simulink model "AirCooledDataCenterTemperatureProfile"  (R2025b)
settings: Solver=daessc  StartTime=0.0  StopTime=24*3600  MaxStep=1  RelTol=1e-3  AbsTol=1e-3
PreLoadFcn:
  | if ~exist("airCooledDataCenter")
  |     setModelParam;
  | end
undefined symbols (not defined in the file or in its folder): airCooledDataCenter, DiscIntNeverNeededParam, value
libraries: fl_lib x166, nesl_utility x25, datacenter_lib x24, simulink_extras x9
(part 2 of 4)

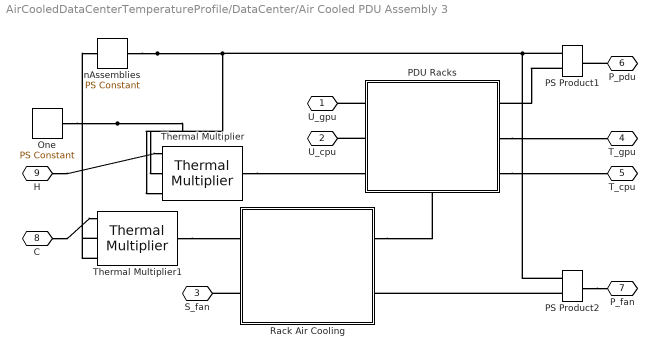
== system AirCooledDataCenterTemperatureProfile/DataCenter/Air Cooled PDU Assembly 3 ==
  One : fl_lib/Physical Signals/Sources/PS Constant  constant=1
  PDU Racks : Subsystem  mask{nTrays=nTrays, nRacks=nRacks, trayMass=trayMass, trayCp=trayCp, trayThermalR=trayThermalR, nGPU=nGPU, gpuTDPperDie=gpuTDPperDie, gpuIdlePower=gpuIdlePower, gpuHBMpower=gpuHBMpower, gpuExponent=gpuExponent, gpuHBMutil=gpuHBMutil, gpuLeakage=gpuLeakage, gpuNominalDieT=gpuNominalDieT, gpuDieThermalC=gpuDieThermalC, gpuHeatSinkR=gpuHeatSinkR, gpuSurfArea=gpuSurfArea, gpuAmbientR=gpuAmbientR, nCPU=nCPU, cpuTDPperSocket=cpuTDPperSocket, cpuIdlePower=cpuIdlePower, cpuExponent=cpuExponent, cpuLeakage=cpuLeakage, cpuNominalDieT=cpuNominalDieT, cpuDieThermalC=cpuDieThermalC, cpuHeatSinkR=cpuHeatSinkR, cpuSurfArea=cpuSurfArea, cpuAmbientR=cpuAmbientR, initialT=initialT, htc=htc}
      mask prompts: nTrays "Number of IT trays per rack (-)"; nRacks "Number of racks (-)"; trayMass "Tray mass (kg)"; trayCp "Tray specific heat capacity (J/kg*K)"; trayThermalR "Tray to external thermal resistance (K/W)"; nGPU "Number of GPU per tray (-)"; gpuTDPperDie "GPU TDP per die (W)"; gpuIdlePower "GPU idle power (W)"; gpuHBMpower "HBM power per GPU (W)"; gpuExponent "GPU power utilization exponent (-)"; gpuHBMutil "HBM utilization as fraction of compute utilization (-)"; gpuLeakage "Leakage increase per K above nominal temperature (W/K)"; gpuNominalDieT "Nominal die temperature at TDP (K)"; gpuDieThermalC "GPU die thermal capacitance (J/K)"; gpuHeatSinkR "GPU die-heat-sink thermal resistance (K/W)"; gpuSurfArea "Surface area per die for ambient heat transfer (m^2)"; gpuAmbientR "GPU die-ambient thermal resistance (K/W)"; nCPU "Number of CPU per tray (-)"; cpuTDPperSocket "CPU TDP per socket (W)"; cpuIdlePower "CPU idle power per socket (W)"; cpuExponent "CPU power utilization exponent (-)"; cpuLeakage "Leakage increase per K above nominal temperature (W/K)"; cpuNominalDieT "Nominal die temperature at TDP (K)"; cpuDieThermalC "CPU die thermal capacitance (J/K)"; cpuHeatSinkR "CPU die-heat-sink thermal resistance (K/W)"; cpuSurfArea "Surface area per die for ambient heat transfer (m^2)"; cpuAmbientR "CPU die-ambient thermal resistance (K/W)"; initialT "Initial temperature (K)"; htc "Heat transfer coefficient to ambient (W/m^2.K)"
      settings: CopyFcn=set_param(gcbh,'LinkStatus','none');  PortSchema="{\"entries\":[{\"content\":{\"sides\":[{\"content\":{\"connectorIds\":[\"LConn1\",\"LConn2\",\"LConn3\"]},\"type\":\"ConnectorPlacement.EquallySpacedRectSide\",\"uuid\":\"1a9a884a-dab1-4495-bf62-c6b2de6c1039\"},{\"content\":{\"connectorIds\":[\"RConn1\",\"RConn2\",\"RConn3\"],\"side\":\"RIGHT\"},\"type\":\"ConnectorPlacement.EquallySpacedRectSide\",\"uuid\":\"05c53434-51c1-4fee-b885-c321dcda8b6b\"},{\"content\":{\"side\":\"TOP\"},\"type\":\"ConnectorPlacement.EquallySpacedRectSide\",\"uuid\":\"c7b5c534-d596-4858-a133-27f005e6c9d4\"},{\"content\":{\"connectorIds\":[\"RConn4\"],\"side\":\"BOTTOM\"},\"type\":\"ConnectorPlacement.EquallySpacedRectSide\",\"uuid\":\"693f3c99-4296-4d86-bfcc-da753d3e576f\"}]},\"type\":\"ConnectorPlacement.EquallySpacedConnector\",\"uuid\":\"ed91c467-c4d0-403f-af16-bac0257594fd\"}],\"packageUris\":[\"http://schema.mathworks.com/mf0/Connector/R2020b\"],\"version\":\"1.0\"}"
      mask Help: web("DocumentationPDURacks.html")
      mask DialogControl Container10 Prompt: PDU Racks
      mask DialogControl getRatingButton Prompt: Get Rating
      mask DialogControl Container9 Prompt: IT Tray
      mask DialogControl Container6 Prompt: GPU
      mask DialogControl Container7 Prompt: CPU
      mask DialogControl Container8 Prompt: Initial Conditions
      mask Display: image('icon_PDURacks.png');
  PS Product1 : fl_lib/Physical Signals/Functions/PS Product
  PS Product2 : fl_lib/Physical Signals/Functions/PS Product
  Rack Air Cooling : Subsystem  mask{nFans=nFans, flowVec=flowVec, prDropVec=prDropVec, fanEffVec=fanEffVec, fluidDen=1.28, fluidCp=1005}
      mask prompts: nFans "Number of fans (-)"; flowVec "Fan flow rate vector (m^3/s)"; prDropVec "Pressure drop vector (Pa)"; fanEffVec "Fan efficiency vector (-)"; fluidDen "Fluid density (kg/m^3)"; fluidCp "Fluid heat capacity (J/(Kg*K))"
      settings: CopyFcn=set_param(gcbh,'LinkStatus','none');
      mask Help: web("DocumentationRackAirCooling.html")
      mask DialogControl Container3 Prompt: Fans
      mask DialogControl Container4 Prompt: Fluid Properties
      mask Display: image('icon_PDUfanCooling.png');
  Thermal Multiplier : datacenter_lib/Thermal Multiplier
      settings: InternalSimscapePortConfiguration="{\"Bottom\":[],\"Left\":[{\"id\":\"A\",\"label\":\"A\",\"type\":\"foundation.thermal.thermal\"}],\"Right\":[{\"id\":\"B\",\"label\":\"B\",\"type\":\"foundation.thermal.thermal\"}],\"Top\":[{\"id\":\"Na\",\"label\":\"Na\",\"type\":\"input\"},{\"id\":\"Nb\",\"label\":\"Nb\",\"type\":\"input\"}]}"
  Thermal Multiplier1 : datacenter_lib/Thermal Multiplier
      settings: InternalSimscapePortConfiguration="{\"Bottom\":[],\"Left\":[{\"id\":\"A\",\"label\":\"A\",\"type\":\"foundation.thermal.thermal\"}],\"Right\":[{\"id\":\"B\",\"label\":\"B\",\"type\":\"foundation.thermal.thermal\"}],\"Top\":[{\"id\":\"Na\",\"label\":\"Na\",\"type\":\"input\"},{\"id\":\"Nb\",\"label\":\"Nb\",\"type\":\"input\"}]}"
  nAssemblies : fl_lib/Physical Signals/Sources/PS Constant  constant=nAssembly
  U_gpu : PMIOPort  Side=Left
  U_cpu : PMIOPort  Port=2  Side=Left
  S_fan : PMIOPort  Port=3  Side=Left
  T_gpu : PMIOPort  Port=4  Side=Right
  T_cpu : PMIOPort  Port=5  Side=Right
  P_pdu : PMIOPort  Port=6  Side=Right
  P_fan : PMIOPort  Port=7  Side=Right
  C : PMIOPort  Port=8  Side=Left
  H : PMIOPort  Port=9  Side=Right
  connections:
  C/RConn1 -- Thermal Multiplier1/LConn1
  H/RConn1 -- Thermal Multiplier/LConn1
  Thermal Multiplier1/RConn1 -- Rack Air Cooling/LConn1
  PS Product2/LConn2 -- Rack Air Cooling/RConn2
  PS Product2/RConn1 -- P_fan/RConn1
  PS Product1/LConn2 -- PDU Racks/RConn1
  P_pdu/RConn1 -- PS Product1/RConn1
  Thermal Multiplier/LConn2 -- Thermal Multiplier1/LConn2 -- One/RConn1
  Thermal Multiplier/LConn3 -- PS Product2/LConn1 -- PS Product1/LConn1 -- Thermal Multiplier1/LConn3 -- nAssemblies/RConn1
  Thermal Multiplier/RConn1 -- PDU Racks/LConn3
  PDU Racks/LConn1 -- U_gpu/RConn1
  Rack Air Cooling/LConn2 -- S_fan/RConn1
  PDU Racks/RConn2 -- T_gpu/RConn1
  PDU Racks/LConn2 -- U_cpu/RConn1
  PDU Racks/RConn3 -- T_cpu/RConn1
  Rack Air Cooling/RConn1 -- PDU Racks/RConn4

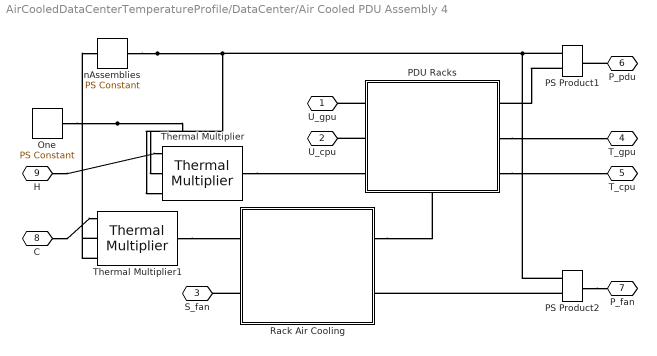
== system AirCooledDataCenterTemperatureProfile/DataCenter/Air Cooled PDU Assembly 4 ==
  One : fl_lib/Physical Signals/Sources/PS Constant  constant=1
  PDU Racks : Subsystem  mask{nTrays=nTrays, nRacks=nRacks, trayMass=trayMass, trayCp=trayCp, trayThermalR=trayThermalR, nGPU=nGPU, gpuTDPperDie=gpuTDPperDie, gpuIdlePower=gpuIdlePower, gpuHBMpower=gpuHBMpower, gpuExponent=gpuExponent, gpuHBMutil=gpuHBMutil, gpuLeakage=gpuLeakage, gpuNominalDieT=gpuNominalDieT, gpuDieThermalC=gpuDieThermalC, gpuHeatSinkR=gpuHeatSinkR, gpuSurfArea=gpuSurfArea, gpuAmbientR=gpuAmbientR, nCPU=nCPU, cpuTDPperSocket=cpuTDPperSocket, cpuIdlePower=cpuIdlePower, cpuExponent=cpuExponent, cpuLeakage=cpuLeakage, cpuNominalDieT=cpuNominalDieT, cpuDieThermalC=cpuDieThermalC, cpuHeatSinkR=cpuHeatSinkR, cpuSurfArea=cpuSurfArea, cpuAmbientR=cpuAmbientR, initialT=initialT, htc=htc}
      mask prompts: nTrays "Number of IT trays per rack (-)"; nRacks "Number of racks (-)"; trayMass "Tray mass (kg)"; trayCp "Tray specific heat capacity (J/kg*K)"; trayThermalR "Tray to external thermal resistance (K/W)"; nGPU "Number of GPU per tray (-)"; gpuTDPperDie "GPU TDP per die (W)"; gpuIdlePower "GPU idle power (W)"; gpuHBMpower "HBM power per GPU (W)"; gpuExponent "GPU power utilization exponent (-)"; gpuHBMutil "HBM utilization as fraction of compute utilization (-)"; gpuLeakage "Leakage increase per K above nominal temperature (W/K)"; gpuNominalDieT "Nominal die temperature at TDP (K)"; gpuDieThermalC "GPU die thermal capacitance (J/K)"; gpuHeatSinkR "GPU die-heat-sink thermal resistance (K/W)"; gpuSurfArea "Surface area per die for ambient heat transfer (m^2)"; gpuAmbientR "GPU die-ambient thermal resistance (K/W)"; nCPU "Number of CPU per tray (-)"; cpuTDPperSocket "CPU TDP per socket (W)"; cpuIdlePower "CPU idle power per socket (W)"; cpuExponent "CPU power utilization exponent (-)"; cpuLeakage "Leakage increase per K above nominal temperature (W/K)"; cpuNominalDieT "Nominal die temperature at TDP (K)"; cpuDieThermalC "CPU die thermal capacitance (J/K)"; cpuHeatSinkR "CPU die-heat-sink thermal resistance (K/W)"; cpuSurfArea "Surface area per die for ambient heat transfer (m^2)"; cpuAmbientR "CPU die-ambient thermal resistance (K/W)"; initialT "Initial temperature (K)"; htc "Heat transfer coefficient to ambient (W/m^2.K)"
      settings: CopyFcn=set_param(gcbh,'LinkStatus','none');  PortSchema="{\"entries\":[{\"content\":{\"sides\":[{\"content\":{\"connectorIds\":[\"LConn1\",\"LConn2\",\"LConn3\"]},\"type\":\"ConnectorPlacement.EquallySpacedRectSide\",\"uuid\":\"1a9a884a-dab1-4495-bf62-c6b2de6c1039\"},{\"content\":{\"connectorIds\":[\"RConn1\",\"RConn2\",\"RConn3\"],\"side\":\"RIGHT\"},\"type\":\"ConnectorPlacement.EquallySpacedRectSide\",\"uuid\":\"05c53434-51c1-4fee-b885-c321dcda8b6b\"},{\"content\":{\"side\":\"TOP\"},\"type\":\"ConnectorPlacement.EquallySpacedRectSide\",\"uuid\":\"c7b5c534-d596-4858-a133-27f005e6c9d4\"},{\"content\":{\"connectorIds\":[\"RConn4\"],\"side\":\"BOTTOM\"},\"type\":\"ConnectorPlacement.EquallySpacedRectSide\",\"uuid\":\"693f3c99-4296-4d86-bfcc-da753d3e576f\"}]},\"type\":\"ConnectorPlacement.EquallySpacedConnector\",\"uuid\":\"ed91c467-c4d0-403f-af16-bac0257594fd\"}],\"packageUris\":[\"http://schema.mathworks.com/mf0/Connector/R2020b\"],\"version\":\"1.0\"}"
      mask Help: web("DocumentationPDURacks.html")
      mask DialogControl Container10 Prompt: PDU Racks
      mask DialogControl getRatingButton Prompt: Get Rating
      mask DialogControl Container9 Prompt: IT Tray
      mask DialogControl Container6 Prompt: GPU
      mask DialogControl Container7 Prompt: CPU
      mask DialogControl Container8 Prompt: Initial Conditions
      mask Display: image('icon_PDURacks.png');
  PS Product1 : fl_lib/Physical Signals/Functions/PS Product
  PS Product2 : fl_lib/Physical Signals/Functions/PS Product
  Rack Air Cooling : Subsystem  mask{nFans=nFans, flowVec=flowVec, prDropVec=prDropVec, fanEffVec=fanEffVec, fluidDen=1.28, fluidCp=1005}
      mask prompts: nFans "Number of fans (-)"; flowVec "Fan flow rate vector (m^3/s)"; prDropVec "Pressure drop vector (Pa)"; fanEffVec "Fan efficiency vector (-)"; fluidDen "Fluid density (kg/m^3)"; fluidCp "Fluid heat capacity (J/(Kg*K))"
      settings: CopyFcn=set_param(gcbh,'LinkStatus','none');
      mask Help: web("DocumentationRackAirCooling.html")
      mask DialogControl Container3 Prompt: Fans
      mask DialogControl Container4 Prompt: Fluid Properties
      mask Display: image('icon_PDUfanCooling.png');
  Thermal Multiplier : datacenter_lib/Thermal Multiplier
      settings: InternalSimscapePortConfiguration="{\"Bottom\":[],\"Left\":[{\"id\":\"A\",\"label\":\"A\",\"type\":\"foundation.thermal.thermal\"}],\"Right\":[{\"id\":\"B\",\"label\":\"B\",\"type\":\"foundation.thermal.thermal\"}],\"Top\":[{\"id\":\"Na\",\"label\":\"Na\",\"type\":\"input\"},{\"id\":\"Nb\",\"label\":\"Nb\",\"type\":\"input\"}]}"
  Thermal Multiplier1 : datacenter_lib/Thermal Multiplier
      settings: InternalSimscapePortConfiguration="{\"Bottom\":[],\"Left\":[{\"id\":\"A\",\"label\":\"A\",\"type\":\"foundation.thermal.thermal\"}],\"Right\":[{\"id\":\"B\",\"label\":\"B\",\"type\":\"foundation.thermal.thermal\"}],\"Top\":[{\"id\":\"Na\",\"label\":\"Na\",\"type\":\"input\"},{\"id\":\"Nb\",\"label\":\"Nb\",\"type\":\"input\"}]}"
  nAssemblies : fl_lib/Physical Signals/Sources/PS Constant  constant=nAssembly
  U_gpu : PMIOPort  Side=Left
  U_cpu : PMIOPort  Port=2  Side=Left
  S_fan : PMIOPort  Port=3  Side=Left
  T_gpu : PMIOPort  Port=4  Side=Right
  T_cpu : PMIOPort  Port=5  Side=Right
  P_pdu : PMIOPort  Port=6  Side=Right
  P_fan : PMIOPort  Port=7  Side=Right
  C : PMIOPort  Port=8  Side=Left
  H : PMIOPort  Port=9  Side=Right
  connections:
  C/RConn1 -- Thermal Multiplier1/LConn1
  H/RConn1 -- Thermal Multiplier/LConn1
  Thermal Multiplier1/RConn1 -- Rack Air Cooling/LConn1
  PS Product2/LConn2 -- Rack Air Cooling/RConn2
  PS Product2/RConn1 -- P_fan/RConn1
  PS Product1/LConn2 -- PDU Racks/RConn1
  P_pdu/RConn1 -- PS Product1/RConn1
  Thermal Multiplier/LConn2 -- Thermal Multiplier1/LConn2 -- One/RConn1
  Thermal Multiplier/LConn3 -- PS Product2/LConn1 -- PS Product1/LConn1 -- Thermal Multiplier1/LConn3 -- nAssemblies/RConn1
  Thermal Multiplier/RConn1 -- PDU Racks/LConn3
  PDU Racks/LConn1 -- U_gpu/RConn1
  Rack Air Cooling/LConn2 -- S_fan/RConn1
  PDU Racks/RConn2 -- T_gpu/RConn1
  PDU Racks/LConn2 -- U_cpu/RConn1
  PDU Racks/RConn3 -- T_cpu/RConn1
  Rack Air Cooling/RConn1 -- PDU Racks/RConn4

== system AirCooledDataCenterTemperatureProfile/DataCenter/Lumped Room ==
  Controlled Temperature Source : fl_lib/Thermal/Thermal Sources/Controlled Temperature Source
  Convective Heat Transfer : fl_lib/Thermal/Thermal Elements/Convective Heat Transfer  thermal_type=foundation.enum.constant_variable.constant  area=len*wid m^2  heat_tr_coeff=htc W/(K*m^2)  min_heat_tr_coeff=1e-3 W/(K*m^2)  T_specify=off  T_priority=None  T=0 K  T_nominal_specify=off  T_nominal_value=1  T_nominal_unit=K  Q_specify=off  Q_priority=None  Q=0 W  Q_nominal_specify=off  Q_nominal_value=1  Q_nominal_unit=W
  Convective Heat Transfer1 : fl_lib/Thermal/Thermal Elements/Convective Heat Transfer  thermal_type=foundation.enum.constant_variable.constant  area=4*2*(len+wid)*hgt*pc/100 m^2  heat_tr_coeff=htc W/(K*m^2)  min_heat_tr_coeff=1e-3 W/(K*m^2)  T_specify=off  T_priority=None  T=0 K  T_nominal_specify=off  T_nominal_value=1  T_nominal_unit=K  Q_specify=off  Q_priority=None  Q=0 W  Q_nominal_specify=off  Q_nominal_value=1  Q_nominal_unit=W
  PS-Simulink Converter16 : nesl_utility/PS-Simulink Converter  PhysicalDomain=network_engine_domain  SubClassName=ps_output  LeftPortType=input  RightPortType=output  PseudoPeriodic=off  Frequencies=[]  VectorFormat=inherit  Unit=inherit  AffineConversion=off
  Room air mass : fl_lib/Thermal/Thermal Elements/Thermal Mass  mass_type=foundation.enum.constant_variable.constant  mass=len*wid*hgt*(1-pc/100)*1.28 kg  sp_heat=1005 J/(K*kg)  mass_min=1e-6 kg  num_ports=foundation.enum.numPorts2.two  m_specify=off  m_priority=High  m=1 kg  m_nominal_specify=off  m_nominal_value=1  m_nominal_unit=kg  T_specify=on  T_priority=High  T=iniT K  T_nominal_specify=off  T_nominal_value=1  T_nominal_unit=K  Q_specify=off  Q_priority=None  Q=0 W  Q_nominal_specify=off  Q_nominal_value=1  Q_nominal_unit=W
      settings: InternalSimscapePortConfiguration="{\"Bottom\":[],\"Left\":[{\"id\":\"M\",\"label\":\"\",\"type\":\"foundation.thermal.thermal\"}],\"Right\":[{\"id\":\"N\",\"label\":\"\",\"type\":\"foundation.thermal.thermal\"}],\"Top\":[]}"
  Temperature Sensor : fl_lib/Thermal/Thermal Sensors/Temperature Sensor  temperature_measure=foundation.enum.MeasurementReference.absolute
      settings: InternalSimscapePortConfiguration="{\"Bottom\":[],\"Left\":[{\"id\":\"A\",\"label\":\"A\",\"type\":\"foundation.thermal.thermal\"}],\"Right\":[{\"id\":\"T\",\"label\":\"T\",\"type\":\"output\"}],\"Top\":[]}"
  Thermal Reference : fl_lib/Thermal/Thermal Elements/Thermal Reference
  Ts : PMIOPort  Side=Left
  C : PMIOPort  Port=2  Side=Left
  H : PMIOPort  Port=3  Side=Right
  Amb : PMIOPort  Port=4  Side=Right
  Tr : Outport
  wires:
  PS-Simulink Converter16/1 -> Tr/1  "Room T"
  connections:
  Temperature Sensor/LConn1 -- Room air mass/LConn1
  Thermal Reference/LConn1 -- Controlled Temperature Source/RConn2
  Temperature Sensor/RConn1 -- Controlled Temperature Source/RConn1 -- PS-Simulink Converter16/LConn1
  Ts/RConn1 -- Convective Heat Transfer/LConn1
  C/RConn1 -- Controlled Temperature Source/LConn1
  Convective Heat Transfer/RConn1 -- Room air mass/RConn1 -- Amb/RConn1 -- Convective Heat Transfer1/LConn1
  Convective Heat Transfer1/RConn1 -- H/RConn1

== system AirCooledDataCenterTemperatureProfile/Fan Speed Control/Subsystem4 ==
  PS Concatenate : fl_lib/Physical Signals/Functions/PS Concatenate  catColumns=true
      settings: InternalSimscapePortConfiguration="{\"Bottom\":[],\"Left\":[{\"id\":\"I1\",\"label\":\"\",\"type\":\"input\"},{\"id\":\"I2\",\"label\":\"\",\"type\":\"input\"}],\"Right\":[{\"id\":\"O\",\"label\":\"\",\"type\":\"output\"}],\"Top\":[]}"
  PS Concatenate1 : fl_lib/Physical Signals/Functions/PS Concatenate  catColumns=true
      settings: InternalSimscapePortConfiguration="{\"Bottom\":[],\"Left\":[{\"id\":\"I1\",\"label\":\"\",\"type\":\"input\"},{\"id\":\"I2\",\"label\":\"\",\"type\":\"input\"}],\"Right\":[{\"id\":\"O\",\"label\":\"\",\"type\":\"output\"}],\"Top\":[]}"
  PS Concatenate2 : fl_lib/Physical Signals/Functions/PS Concatenate  catColumns=true
      settings: InternalSimscapePortConfiguration="{\"Bottom\":[],\"Left\":[{\"id\":\"I1\",\"label\":\"\",\"type\":\"input\"},{\"id\":\"I2\",\"label\":\"\",\"type\":\"input\"}],\"Right\":[{\"id\":\"O\",\"label\":\"\",\"type\":\"output\"}],\"Top\":[]}"
  S4 : PMIOPort  Side=Left
  S3 : PMIOPort  Port=2  Side=Left
  S2 : PMIOPort  Port=3  Side=Left
  S1 : PMIOPort  Port=4  Side=Left
  F : PMIOPort  Port=5  Side=Right
  connections:
  PS Concatenate2/LConn2 -- S4/RConn1
  PS Concatenate/LConn2 -- S2/RConn1
  PS Concatenate1/LConn1 -- PS Concatenate/RConn1
  PS Concatenate2/LConn1 -- PS Concatenate1/RConn1
  PS Concatenate1/LConn2 -- S3/RConn1
  F/RConn1 -- PS Concatenate2/RConn1
  PS Concatenate/LConn1 -- S1/RConn1

== system AirCooledDataCenterTemperatureProfile/Fan Speed Control/Subsystem5 ==
  T : Inport
  D1 : BusSelector  OutputSignals=D1.Max,D1.Min
  D2 : BusSelector  OutputSignals=D2.Max,D2.Min
  D3 : BusSelector  OutputSignals=D3.Max,D3.Min
  D4 : BusSelector  OutputSignals=D4.Max,D4.Min
  Subsystem : Subsystem  mask{Ts=measDelay, uppT=upperT, lowT=lowerT}
      mask prompts: Ts "Measurement delay (s)"; uppT "Upper limit temperature (K)"; lowT "Lower limit temperature (K)"
      settings: PortSchema="{\"entries\":[{\"content\":{\"sides\":[{\"content\":{\"connectorIds\":[\"LConn1\"]},\"type\":\"ConnectorPlacement.EquallySpacedRectSide\",\"uuid\":\"76a0f47d-e2da-464e-af47-d1de2c0a2775\"},{\"content\":{\"connectorIds\":[\"In1\",\"In2\"],\"side\":\"RIGHT\"},\"type\":\"ConnectorPlacement.EquallySpacedRectSide\",\"uuid\":\"4720b8d8-bdaf-4068-88d8-7e817175b798\"},{\"content\":{\"side\":\"TOP\"},\"type\":\"ConnectorPlacement.EquallySpacedRectSide\",\"uuid\":\"0c4cf0ed-7be6-4add-afae-556b60096d13\"}]},\"type\":\"ConnectorPlacement.EquallySpacedConnector\",\"uuid\":\"5d672270-c8d8-4cc8-adff-c30d9f578126\"}],\"packageUris\":[\"http://schema.mathworks.com/mf0/Connector/R2020b\"],\"version\":\"1.0\"}"
  Subsystem1 : Subsystem  mask{Ts=measDelay, uppT=upperT, lowT=lowerT}
      mask prompts: Ts "Measurement delay (s)"; uppT "Upper limit temperature (K)"; lowT "Lower limit temperature (K)"
      settings: PortSchema="{\"entries\":[{\"content\":{\"sides\":[{\"content\":{\"connectorIds\":[\"LConn1\"]},\"type\":\"ConnectorPlacement.EquallySpacedRectSide\",\"uuid\":\"76a0f47d-e2da-464e-af47-d1de2c0a2775\"},{\"content\":{\"connectorIds\":[\"In1\",\"In2\"],\"side\":\"RIGHT\"},\"type\":\"ConnectorPlacement.EquallySpacedRectSide\",\"uuid\":\"4720b8d8-bdaf-4068-88d8-7e817175b798\"},{\"content\":{\"side\":\"TOP\"},\"type\":\"ConnectorPlacement.EquallySpacedRectSide\",\"uuid\":\"0c4cf0ed-7be6-4add-afae-556b60096d13\"}]},\"type\":\"ConnectorPlacement.EquallySpacedConnector\",\"uuid\":\"5d672270-c8d8-4cc8-adff-c30d9f578126\"}],\"packageUris\":[\"http://schema.mathworks.com/mf0/Connector/R2020b\"],\"version\":\"1.0\"}"
  Subsystem2 : Subsystem  mask{Ts=measDelay, uppT=upperT, lowT=lowerT}
      mask prompts: Ts "Measurement delay (s)"; uppT "Upper limit temperature (K)"; lowT "Lower limit temperature (K)"
      settings: PortSchema="{\"entries\":[{\"content\":{\"sides\":[{\"content\":{\"connectorIds\":[\"LConn1\"]},\"type\":\"ConnectorPlacement.EquallySpacedRectSide\",\"uuid\":\"76a0f47d-e2da-464e-af47-d1de2c0a2775\"},{\"content\":{\"connectorIds\":[\"In1\",\"In2\"],\"side\":\"RIGHT\"},\"type\":\"ConnectorPlacement.EquallySpacedRectSide\",\"uuid\":\"4720b8d8-bdaf-4068-88d8-7e817175b798\"},{\"content\":{\"side\":\"TOP\"},\"type\":\"ConnectorPlacement.EquallySpacedRectSide\",\"uuid\":\"0c4cf0ed-7be6-4add-afae-556b60096d13\"}]},\"type\":\"ConnectorPlacement.EquallySpacedConnector\",\"uuid\":\"5d672270-c8d8-4cc8-adff-c30d9f578126\"}],\"packageUris\":[\"http://schema.mathworks.com/mf0/Connector/R2020b\"],\"version\":\"1.0\"}"
  Subsystem3 : Subsystem  mask{Ts=measDelay, uppT=upperT, lowT=lowerT}
      mask prompts: Ts "Measurement delay (s)"; uppT "Upper limit temperature (K)"; lowT "Lower limit temperature (K)"
      settings: PortSchema="{\"entries\":[{\"content\":{\"sides\":[{\"content\":{\"connectorIds\":[\"LConn1\"]},\"type\":\"ConnectorPlacement.EquallySpacedRectSide\",\"uuid\":\"76a0f47d-e2da-464e-af47-d1de2c0a2775\"},{\"content\":{\"connectorIds\":[\"In1\",\"In2\"],\"side\":\"RIGHT\"},\"type\":\"ConnectorPlacement.EquallySpacedRectSide\",\"uuid\":\"4720b8d8-bdaf-4068-88d8-7e817175b798\"},{\"content\":{\"side\":\"TOP\"},\"type\":\"ConnectorPlacement.EquallySpacedRectSide\",\"uuid\":\"0c4cf0ed-7be6-4add-afae-556b60096d13\"}]},\"type\":\"ConnectorPlacement.EquallySpacedConnector\",\"uuid\":\"5d672270-c8d8-4cc8-adff-c30d9f578126\"}],\"packageUris\":[\"http://schema.mathworks.com/mf0/Connector/R2020b\"],\"version\":\"1.0\"}"
  S1 : PMIOPort  Side=Left
  S2 : PMIOPort  Port=2  Side=Left
  S3 : PMIOPort  Port=3  Side=Left
  S4 : PMIOPort  Port=4  Side=Left
  wires:
  D2/1 -> Subsystem1/1(<Max>)  "<Max>"
  D4/1 -> Subsystem3/1(<Max>)  "<Max>"
  D4/2 -> Subsystem3/2(<Min>)  "<Min>"
  D3/1 -> Subsystem2/1(<Max>)  "<Max>"
  D2/2 -> Subsystem1/2(<Min>)  "<Min>"
  D1/1 -> Subsystem/1(<Max>)  "<Max>"
  D1/2 -> Subsystem/2(<Min>)  "<Min>"
  D3/2 -> Subsystem2/2(<Min>)  "<Min>"
  T/1 -> D4/1, D3/1, D2/1, D1/1
  connections:
  Subsystem2/LConn1 -- S3/RConn1
  Subsystem3/LConn1 -- S4/RConn1
  S1/RConn1 -- Subsystem/LConn1
  Subsystem1/LConn1 -- S2/RConn1

== system AirCooledDataCenterTemperatureProfile/Room HVAC Control/Room HVAC ==
  Tr : Inport
  Ts : Inport  Port=2
  Abs : Abs  SaturateOnIntegerOverflow=off
  Bus Creator : BusCreator  Inputs=2
  Constant2 : Constant  Value=effHeatExchanger/100
  Transfer Fcn (with initial outputs) : simulink_extras/Additional Linear/Transfer Fcn (with initial outputs)  N=[1]  D="[1  tLag]"  Y0=1  U0=0
  air Cp : Constant  Value=1005
  deltaT : Sum  Inputs=+-
  ePower : Product  Inputs=*/
  m_dot_Cp times deltaT : Product  Inputs=3
  mass room air volume : Constant  Value=roomLen*roomWid*roomHt*(1-fracRoomVolDC)*1.28
  S : Outport
  wires:
  Ts/1 -> deltaT/1
  deltaT/1 -> m_dot_Cp times deltaT/3
  Tr/1 -> deltaT/2
  Constant2/1 -> ePower/2
  ePower/1 -> Abs/1
  air Cp/1 -> m_dot_Cp times deltaT/1
  mass room air volume/1 -> m_dot_Cp times deltaT/2
  Abs/1 -> Bus Creator/2  "P"
  Bus Creator/1 -> S/1  "hvac"
  Transfer Fcn (with initial outputs)/1 -> Bus Creator/1, ePower/1  "Q"
  m_dot_Cp times deltaT/1 -> Transfer Fcn (with initial outputs)/1  "Q"

== system AirCooledDataCenterTemperatureProfile/Room HVAC Control/Subsystem ==
  S : Inport
  Bus Selector : BusSelector  OutputSignals=Q,P
  Controlled Heat Flow Rate Source : fl_lib/Thermal/Thermal Sources/Controlled Heat Flow Rate Source
  Simulink-PS Converter : nesl_utility/Simulink-PS Converter  PhysicalDomain=network_engine_domain  SubClassName=ps_input  LeftPortType=input  RightPortType=output  PseudoPeriodic=off  Frequencies=[]  NoiseDistribution=none  NoiseParameters=[]  Unit=J/s  AffineConversion=off  FilteringAndDerivatives=provide  SimscapeFilterOrder=1  InputFilterTimeConstant=0.001  UdotUserProvided=0
  Thermal Reference : fl_lib/Thermal/Thermal Elements/Thermal Reference
  C : PMIOPort  Side=Right
  P : Outport
  wires:
  Bus Selector/1 -> Simulink-PS Converter/1  "<Q>"
  S/1 -> Bus Selector/1
  Bus Selector/2 -> P/1  "<P>"
  connections:
  Simulink-PS Converter/RConn1 -- Controlled Heat Flow Rate Source/RConn1
  Thermal Reference/LConn1 -- Controlled Heat Flow Rate Source/RConn2
  Controlled Heat Flow Rate Source/LConn1 -- C/RConn1

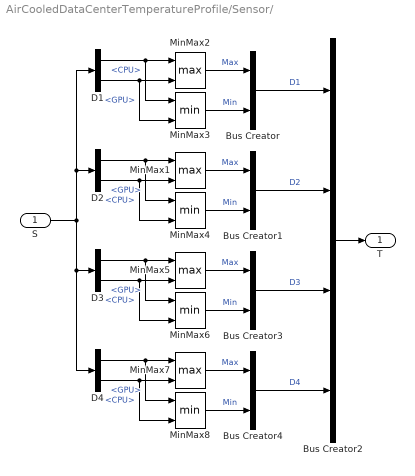
== system AirCooledDataCenterTemperatureProfile/Sensor/  ==
  S : Inport
  Bus Creator{,1,3..4} (4 alike) : BusCreator  Inputs=2
  Bus Creator2 : BusCreator  Inputs=4
  D1 : BusSelector  OutputSignals=D1.CPU,D1.GPU
  D2 : BusSelector  OutputSignals=D2.GPU,D2.CPU
  D3 : BusSelector  OutputSignals=D3.GPU,D3.CPU
  D4 : BusSelector  OutputSignals=D4.GPU,D4.CPU
  MinMax{1..2,5,7} (4 alike) : MinMax  Function=max  Inputs=2
  MinMax{3..4,6,8} (4 alike) : MinMax  Inputs=2
  T : Outport
  wires:
  D1/2 -> MinMax3/2, MinMax2/2  "<GPU>"
  D1/1 -> MinMax3/1, MinMax2/1  "<CPU>"
  MinMax2/1 -> Bus Creator/1  "Max"
  MinMax3/1 -> Bus Creator/2  "Min"
  D2/1 -> MinMax4/1, MinMax1/1  "<GPU>"
  MinMax4/1 -> Bus Creator1/2  "Min"
  D2/2 -> MinMax4/2, MinMax1/2  "<CPU>"
  MinMax1/1 -> Bus Creator1/1  "Max"
  Bus Creator/1 -> Bus Creator2/1  "D1"
  Bus Creator1/1 -> Bus Creator2/2  "D2"
  Bus Creator2/1 -> T/1
  MinMax5/1 -> Bus Creator3/1  "Max"
  MinMax6/1 -> Bus Creator3/2  "Min"
  D3/2 -> MinMax6/2, MinMax5/2  "<CPU>"
  Bus Creator3/1 -> Bus Creator2/3  "D3"
  D3/1 -> MinMax6/1, MinMax5/1  "<GPU>"
  MinMax7/1 -> Bus Creator4/1  "Max"
  MinMax8/1 -> Bus Creator4/2  "Min"
  D4/2 -> MinMax8/2, MinMax7/2  "<CPU>"
  Bus Creator4/1 -> Bus Creator2/4  "D4"
  S/1 -> D1/1, D2/1, D4/1, D3/1
  D4/1 -> MinMax8/1, MinMax7/1  "<GPU>"

== system AirCooledDataCenterTemperatureProfile/Sensor/Subsystem2 ==
  S : Inport
  Discrete-Time Integrator : DiscreteIntegrator  gainval=1  InitialCondition=1  SampleTime=sampleTimeSec  ICPrevOutput=DiscIntNeverNeededParam  ICPrevScaledInput=DiscIntNeverNeededParam
  Divide : Product  Inputs=*/
  Subsystem : Subsystem
  R : Outport
  wires:
  Discrete-Time Integrator/1 -> Divide/1
  Subsystem/1(" ") -> Divide/2
  S/1 -> Discrete-Time Integrator/1
  Divide/1 -> R/1

== system AirCooledDataCenterTemperatureProfile/Sensor/Subsystem3 ==
  S : Inport
  Discrete-Time Integrator : DiscreteIntegrator  gainval=1  InitialCondition=1  SampleTime=sampleTimeSec  ICPrevOutput=DiscIntNeverNeededParam  ICPrevScaledInput=DiscIntNeverNeededParam
  Divide : Product  Inputs=*/
  Subsystem : Subsystem
  R : Outport
  wires:
  Discrete-Time Integrator/1 -> Divide/1
  Subsystem/1(" ") -> Divide/2
  S/1 -> Discrete-Time Integrator/1
  Divide/1 -> R/1

== system AirCooledDataCenterTemperatureProfile/Sensor/Subsystem4 ==
  S : Inport
  Discrete-Time Integrator : DiscreteIntegrator  gainval=1  InitialCondition=1  SampleTime=sampleTimeSec  ICPrevOutput=DiscIntNeverNeededParam  ICPrevScaledInput=DiscIntNeverNeededParam
  Divide : Product  Inputs=*/
  Subsystem : Subsystem
  R : Outport
  wires:
  Discrete-Time Integrator/1 -> Divide/1
  Subsystem/1(" ") -> Divide/2
  S/1 -> Discrete-Time Integrator/1
  Divide/1 -> R/1

== system AirCooledDataCenterTemperatureProfile/Uvec/Subsystem ==
  PS Concatenate : fl_lib/Physical Signals/Functions/PS Concatenate  catColumns=true
      settings: InternalSimscapePortConfiguration="{\"Bottom\":[],\"Left\":[{\"id\":\"I1\",\"label\":\"\",\"type\":\"input\"},{\"id\":\"I2\",\"label\":\"\",\"type\":\"input\"}],\"Right\":[{\"id\":\"O\",\"label\":\"\",\"type\":\"output\"}],\"Top\":[]}"
  PS Concatenate1 : fl_lib/Physical Signals/Functions/PS Concatenate  catColumns=true
      settings: InternalSimscapePortConfiguration="{\"Bottom\":[],\"Left\":[{\"id\":\"I1\",\"label\":\"\",\"type\":\"input\"},{\"id\":\"I2\",\"label\":\"\",\"type\":\"input\"}],\"Right\":[{\"id\":\"O\",\"label\":\"\",\"type\":\"output\"}],\"Top\":[]}"
  PS Concatenate2 : fl_lib/Physical Signals/Functions/PS Concatenate  catColumns=true
      settings: InternalSimscapePortConfiguration="{\"Bottom\":[],\"Left\":[{\"id\":\"I1\",\"label\":\"\",\"type\":\"input\"},{\"id\":\"I2\",\"label\":\"\",\"type\":\"input\"}],\"Right\":[{\"id\":\"O\",\"label\":\"\",\"type\":\"output\"}],\"Top\":[]}"
  Conn1 : PMIOPort  Side=Left
  Conn2 : PMIOPort  Port=2  Side=Left
  Conn3 : PMIOPort  Port=3  Side=Right
  Conn4 : PMIOPort  Port=4  Side=Left
  Conn5 : PMIOPort  Port=5  Side=Left
  connections:
  PS Concatenate2/LConn2 -- Conn5/RConn1
  PS Concatenate/LConn2 -- Conn2/RConn1
  PS Concatenate1/LConn1 -- PS Concatenate/RConn1
  PS Concatenate2/LConn1 -- PS Concatenate1/RConn1
  PS Concatenate1/LConn2 -- Conn4/RConn1
  Conn3/RConn1 -- PS Concatenate2/RConn1
  PS Concatenate/LConn1 -- Conn1/RConn1

== system AirCooledDataCenterTemperatureProfile/DataCenter/Air Cooled PDU Assembly 1/PDU Racks ==
  PS Product : fl_lib/Physical Signals/Functions/PS Product
  Server Tray : Subsystem  mask{nGPU=nGPU, gpuTDPperDie=gpuTDPperDie, gpuIdlePower=gpuIdlePower, gpuHBMpower=gpuHBMpower, gpuExponent=gpuExponent, gpuHBMutil=gpuHBMutil, gpuLeakage=gpuLeakage, gpuNominalDieT=gpuNominalDieT, gpuDieThermalC=gpuDieThermalC, gpuHeatSinkR=gpuHeatSinkR, gpuSurfArea=gpuSurfArea, gpuAmbientR=gpuAmbientR, nCPU=nCPU, cpuTDPperSocket=cpuTDPperSocket, cpuIdlePower=cpuIdlePower, cpuExponent=cpuExponent, cpuLeakage=cpuLeakage, cpuNominalDieT=cpuNominalDieT, cpuDieThermalC=cpuDieThermalC, cpuHeatSinkR=cpuHeatSinkR, cpuSurfArea=cpuSurfArea, cpuAmbientR=cpuAmbientR, trayMass=trayMass, trayCp=trayCp, trayThermalR=trayThermalR, initialT=initialT, htc=htc}
      mask prompts: nGPU "Number of GPU (-)"; gpuTDPperDie "GPU TDP per die (W)"; gpuIdlePower "GPU idle power (W)"; gpuHBMpower "HBM power per GPU (W)"; gpuExponent "GPU power utilization exponent (-)"; gpuHBMutil "HBM utilization as fraction of compute utilization (-)"; gpuLeakage "Leakage increase per K above nominal temperature (W/K)"; gpuNominalDieT "Nominal die temperature at TDP (K)"; gpuDieThermalC "GPU die thermal capacitance (J/K)"; gpuHeatSinkR "GPU die-heat-sink thermal resistance (K/W)"; gpuSurfArea "Surface area per die for ambient heat transfer (m^2)"; gpuAmbientR "GPU die-ambient thermal resistance (K/W)"; nCPU "Number of CPU (-)"; cpuTDPperSocket "CPU TDP per socket (W)"; cpuIdlePower "CPU idle power per socket (W)"; cpuExponent "CPU power utilization exponent (-)"; cpuLeakage "Leakage increase per K above nominal temperature (W/K)"; cpuNominalDieT "Nominal die temperature at TDP (K)"; cpuDieThermalC "CPU die thermal capacitance (J/K)"; cpuHeatSinkR "CPU die-heat-sink thermal resistance (K/W)"; cpuSurfArea "Surface area per die for ambient heat transfer (m^2)"; cpuAmbientR "CPU die-ambient thermal resistance (K/W)"; trayMass "Tray mass (kg)"; trayCp "Tray specific heat capacity (J/kg*K)"; trayThermalR "Tray to external thermal resistance (K/W)"; initialT "Initial temperature (K)"; htc "Heat transfer coefficient to ambient (W/m^2.K)"
      settings: CopyFcn=set_param(gcbh,'LinkStatus','none');  PortSchema="{\"entries\":[{\"content\":{\"sides\":[{\"content\":{\"connectorIds\":[\"LConn1\",\"LConn2\",\"LConn3\"]},\"type\":\"ConnectorPlacement.EquallySpacedRectSide\",\"uuid\":\"893f21b9-92d6-433a-96e5-f8193a696c29\"},{\"content\":{\"connectorIds\":[\"RConn1\",\"RConn2\",\"RConn3\"],\"side\":\"RIGHT\"},\"type\":\"ConnectorPlacement.EquallySpacedRectSide\",\"uuid\":\"efd10409-70d8-4a6a-97a2-13f0e6f538e3\"},{\"content\":{\"side\":\"TOP\"},\"type\":\"ConnectorPlacement.EquallySpacedRectSide\",\"uuid\":\"8c9765cd-90e6-46de-916c-606bbb93143e\"},{\"content\":{\"connectorIds\":[\"RConn4\"],\"side\":\"BOTTOM\"},\"type\":\"ConnectorPlacement.EquallySpacedRectSide\",\"uuid\":\"9656b44e-d582-43b0-a7fe-c629821d6c27\"}]},\"type\":\"ConnectorPlacement.EquallySpacedConnector\",\"uuid\":\"add7a682-eb4b-4f46-a5b9-e161ccf96de5\"}],\"packageUris\":[\"http://schema.mathworks.com/mf0/Connector/R2020b\"],\"version\":\"1.0\"}"
      mask Help: web("DocumentationServerTray.html")
      mask DialogControl Container6 Prompt: GPU
      mask DialogControl Container7 Prompt: CPU
      mask DialogControl Container9 Prompt: IT Tray
      mask DialogControl Container8 Prompt: Initial Conditions
      mask Display: image('icon_serverPlate.png');
  TMamb : datacenter_lib/Thermal Multiplier
      settings: InternalSimscapePortConfiguration="{\"Bottom\":[],\"Left\":[{\"id\":\"A\",\"label\":\"A\",\"type\":\"foundation.thermal.thermal\"}],\"Right\":[{\"id\":\"B\",\"label\":\"B\",\"type\":\"foundation.thermal.thermal\"}],\"Top\":[{\"id\":\"Na\",\"label\":\"Na\",\"type\":\"input\"},{\"id\":\"Nb\",\"label\":\"Nb\",\"type\":\"input\"}]}"
  TMcdu : datacenter_lib/Thermal Multiplier
      settings: InternalSimscapePortConfiguration="{\"Bottom\":[],\"Left\":[{\"id\":\"A\",\"label\":\"A\",\"type\":\"foundation.thermal.thermal\"}],\"Right\":[{\"id\":\"B\",\"label\":\"B\",\"type\":\"foundation.thermal.thermal\"}],\"Top\":[{\"id\":\"Na\",\"label\":\"Na\",\"type\":\"input\"},{\"id\":\"Nb\",\"label\":\"Nb\",\"type\":\"input\"}]}"
  nTraysXnRacks : fl_lib/Physical Signals/Sources/PS Constant  constant=nTrays*nRacks
  one : fl_lib/Physical Signals/Sources/PS Constant  constant=1
  U_gpu : PMIOPort  Side=Left
  U_cpu : PMIOPort  Port=2  Side=Left
  Ha : PMIOPort  Port=3  Side=Left
  P : PMIOPort  Port=4  Side=Right
  T_gpu : PMIOPort  Port=5  Side=Right
  T_cpu : PMIOPort  Port=6  Side=Right
  Hc : PMIOPort  Port=7  Side=Right
  connections:
  Server Tray/LConn1 -- U_gpu/RConn1
  TMamb/LConn1 -- Ha/RConn1
  Server Tray/RConn2 -- T_gpu/RConn1
  TMcdu/RConn1 -- Hc/RConn1
  Server Tray/LConn2 -- U_cpu/RConn1
  Server Tray/RConn3 -- T_cpu/RConn1
  one/RConn1 -- TMcdu/LConn3 -- TMamb/LConn2
  Server Tray/RConn4 -- TMcdu/LConn1
  Server Tray/LConn3 -- TMamb/RConn1
  nTraysXnRacks/RConn1 -- PS Product/LConn1 -- TMcdu/LConn2 -- TMamb/LConn3
  Server Tray/RConn1 -- PS Product/LConn2
  PS Product/RConn1 -- P/RConn1

== system AirCooledDataCenterTemperatureProfile/DataCenter/Air Cooled PDU Assembly 1/Rack Air Cooling ==
  Flowrate vs Eff : fl_lib/Physical Signals/Lookup Tables/PS Lookup Table (1D)  x=flowVec m^3/s  f=fanEffVec  interp_method=simscape.enum.interpolation.linear  extrap_method=simscape.enum.extrapolation.nearest
  Flowrate vs Pressure Drop : fl_lib/Physical Signals/Lookup Tables/PS Lookup Table (1D)  x=flowVec m^3/s  f=prDropVec Pa  interp_method=simscape.enum.interpolation.linear  extrap_method=simscape.enum.extrapolation.nearest
  MaxFlowrate : fl_lib/Physical Signals/Functions/PS Gain  gain=max(flowVec) m^3/s
  PS Divide : fl_lib/Physical Signals/Functions/PS Divide
  PS Product : fl_lib/Physical Signals/Functions/PS Product
  PS Product1 : fl_lib/Physical Signals/Functions/PS Product
  PS Saturation : fl_lib/Physical Signals/Nonlinear Operators/PS Saturation  upper_limit=1  lower_limit=0  ZeroCross=true
  Q : Subsystem
  dT : Subsystem
      settings: PortSchema="{\"entries\":[{\"content\":{\"sides\":[{\"content\":{\"connectorIds\":[\"LConn1\"]},\"type\":\"ConnectorPlacement.EquallySpacedRectSide\",\"uuid\":\"24179a54-9ef9-408d-b9e3-71fcbe48c3e7\"},{\"content\":{\"connectorIds\":[\"RConn1\"],\"side\":\"RIGHT\"},\"type\":\"ConnectorPlacement.EquallySpacedRectSide\",\"uuid\":\"9ef8b705-2d29-4693-9aa8-2fb03fb72ba0\"},{\"content\":{\"side\":\"TOP\"},\"type\":\"ConnectorPlacement.EquallySpacedRectSide\",\"uuid\":\"67fd6558-0b74-41b6-9065-c50d20bb7de5\"},{\"content\":{\"connectorIds\":[\"RConn2\"],\"side\":\"BOTTOM\"},\"type\":\"ConnectorPlacement.EquallySpacedRectSide\",\"uuid\":\"dead0843-c913-4c5f-8840-2a92db603c86\"}]},\"type\":\"ConnectorPlacement.EquallySpacedConnector\",\"uuid\":\"734a32c8-d564-4672-86f6-d3d1b9b4eb6d\"}],\"packageUris\":[\"http://schema.mathworks.com/mf0/Connector/R2020b\"],\"version\":\"1.0\"}"
  m_dot_Cp : Subsystem
      settings: PortSchema="{\"entries\":[{\"content\":{\"sides\":[{\"content\":{},\"type\":\"ConnectorPlacement.EquallySpacedRectSide\",\"uuid\":\"30dae9bf-ed85-460d-bbc0-602f54b59459\"},{\"content\":{\"side\":\"RIGHT\"},\"type\":\"ConnectorPlacement.EquallySpacedRectSide\",\"uuid\":\"05907a20-db7b-437b-af9c-28a9e12dbb0f\"},{\"content\":{\"connectorIds\":[\"LConn1\"],\"side\":\"TOP\"},\"type\":\"ConnectorPlacement.EquallySpacedRectSide\",\"uuid\":\"1394250d-0f3a-4d32-aa79-d5be723ed221\"},{\"content\":{\"connectorIds\":[\"RConn1\"],\"side\":\"BOTTOM\"},\"type\":\"ConnectorPlacement.EquallySpacedRectSide\",\"uuid\":\"8d71629e-6ed3-4a45-8875-f0ad6e4187c2\"}]},\"type\":\"ConnectorPlacement.EquallySpacedConnector\",\"uuid\":\"77e9989b-961e-42ca-a28b-c98959ddb965\"}],\"packageUris\":[\"http://schema.mathworks.com/mf0/Connector/R2020b\"],\"version\":\"1.0\"}"
  numFans : fl_lib/Physical Signals/Sources/PS Constant  constant=nFans
  C : PMIOPort  Side=Left
  S : PMIOPort  Port=2  Side=Left
  H : PMIOPort  Port=3  Side=Right
  P : PMIOPort  Port=4  Side=Right
  connections:
  Flowrate vs Eff/LConn1 -- PS Product/LConn2 -- Flowrate vs Pressure Drop/LConn1 -- MaxFlowrate/RConn1 -- m_dot_Cp/RConn1
  PS Product1/LConn2 -- PS Product/RConn1
  PS Saturation/LConn1 -- S/RConn1
  PS Product1/RConn1 -- PS Divide/LConn1
  PS Divide/LConn2 -- Flowrate vs Eff/RConn1
  PS Divide/RConn1 -- P/RConn1
  PS Saturation/RConn1 -- MaxFlowrate/LConn1
  numFans/RConn1 -- PS Product1/LConn1
  PS Product/LConn1 -- Flowrate vs Pressure Drop/RConn1
  Q/RConn1 -- dT/RConn1 -- H/RConn1
  dT/LConn1 -- C/RConn1
  Q/LConn1 -- dT/RConn2
  m_dot_Cp/LConn1 -- Q/LConn2

== system AirCooledDataCenterTemperatureProfile/DataCenter/Air Cooled PDU Assembly 2/PDU Racks ==
  PS Product : fl_lib/Physical Signals/Functions/PS Product
  Server Tray : Subsystem  mask{nGPU=nGPU, gpuTDPperDie=gpuTDPperDie, gpuIdlePower=gpuIdlePower, gpuHBMpower=gpuHBMpower, gpuExponent=gpuExponent, gpuHBMutil=gpuHBMutil, gpuLeakage=gpuLeakage, gpuNominalDieT=gpuNominalDieT, gpuDieThermalC=gpuDieThermalC, gpuHeatSinkR=gpuHeatSinkR, gpuSurfArea=gpuSurfArea, gpuAmbientR=gpuAmbientR, nCPU=nCPU, cpuTDPperSocket=cpuTDPperSocket, cpuIdlePower=cpuIdlePower, cpuExponent=cpuExponent, cpuLeakage=cpuLeakage, cpuNominalDieT=cpuNominalDieT, cpuDieThermalC=cpuDieThermalC, cpuHeatSinkR=cpuHeatSinkR, cpuSurfArea=cpuSurfArea, cpuAmbientR=cpuAmbientR, trayMass=trayMass, trayCp=trayCp, trayThermalR=trayThermalR, initialT=initialT, htc=htc}
      mask prompts: nGPU "Number of GPU (-)"; gpuTDPperDie "GPU TDP per die (W)"; gpuIdlePower "GPU idle power (W)"; gpuHBMpower "HBM power per GPU (W)"; gpuExponent "GPU power utilization exponent (-)"; gpuHBMutil "HBM utilization as fraction of compute utilization (-)"; gpuLeakage "Leakage increase per K above nominal temperature (W/K)"; gpuNominalDieT "Nominal die temperature at TDP (K)"; gpuDieThermalC "GPU die thermal capacitance (J/K)"; gpuHeatSinkR "GPU die-heat-sink thermal resistance (K/W)"; gpuSurfArea "Surface area per die for ambient heat transfer (m^2)"; gpuAmbientR "GPU die-ambient thermal resistance (K/W)"; nCPU "Number of CPU (-)"; cpuTDPperSocket "CPU TDP per socket (W)"; cpuIdlePower "CPU idle power per socket (W)"; cpuExponent "CPU power utilization exponent (-)"; cpuLeakage "Leakage increase per K above nominal temperature (W/K)"; cpuNominalDieT "Nominal die temperature at TDP (K)"; cpuDieThermalC "CPU die thermal capacitance (J/K)"; cpuHeatSinkR "CPU die-heat-sink thermal resistance (K/W)"; cpuSurfArea "Surface area per die for ambient heat transfer (m^2)"; cpuAmbientR "CPU die-ambient thermal resistance (K/W)"; trayMass "Tray mass (kg)"; trayCp "Tray specific heat capacity (J/kg*K)"; trayThermalR "Tray to external thermal resistance (K/W)"; initialT "Initial temperature (K)"; htc "Heat transfer coefficient to ambient (W/m^2.K)"
      settings: CopyFcn=set_param(gcbh,'LinkStatus','none');  PortSchema="{\"entries\":[{\"content\":{\"sides\":[{\"content\":{\"connectorIds\":[\"LConn1\",\"LConn2\",\"LConn3\"]},\"type\":\"ConnectorPlacement.EquallySpacedRectSide\",\"uuid\":\"893f21b9-92d6-433a-96e5-f8193a696c29\"},{\"content\":{\"connectorIds\":[\"RConn1\",\"RConn2\",\"RConn3\"],\"side\":\"RIGHT\"},\"type\":\"ConnectorPlacement.EquallySpacedRectSide\",\"uuid\":\"efd10409-70d8-4a6a-97a2-13f0e6f538e3\"},{\"content\":{\"side\":\"TOP\"},\"type\":\"ConnectorPlacement.EquallySpacedRectSide\",\"uuid\":\"8c9765cd-90e6-46de-916c-606bbb93143e\"},{\"content\":{\"connectorIds\":[\"RConn4\"],\"side\":\"BOTTOM\"},\"type\":\"ConnectorPlacement.EquallySpacedRectSide\",\"uuid\":\"9656b44e-d582-43b0-a7fe-c629821d6c27\"}]},\"type\":\"ConnectorPlacement.EquallySpacedConnector\",\"uuid\":\"add7a682-eb4b-4f46-a5b9-e161ccf96de5\"}],\"packageUris\":[\"http://schema.mathworks.com/mf0/Connector/R2020b\"],\"version\":\"1.0\"}"
      mask Help: web("DocumentationServerTray.html")
      mask DialogControl Container6 Prompt: GPU
      mask DialogControl Container7 Prompt: CPU
      mask DialogControl Container9 Prompt: IT Tray
      mask DialogControl Container8 Prompt: Initial Conditions
      mask Display: image('icon_serverPlate.png');
  TMamb : datacenter_lib/Thermal Multiplier
      settings: InternalSimscapePortConfiguration="{\"Bottom\":[],\"Left\":[{\"id\":\"A\",\"label\":\"A\",\"type\":\"foundation.thermal.thermal\"}],\"Right\":[{\"id\":\"B\",\"label\":\"B\",\"type\":\"foundation.thermal.thermal\"}],\"Top\":[{\"id\":\"Na\",\"label\":\"Na\",\"type\":\"input\"},{\"id\":\"Nb\",\"label\":\"Nb\",\"type\":\"input\"}]}"
  TMcdu : datacenter_lib/Thermal Multiplier
      settings: InternalSimscapePortConfiguration="{\"Bottom\":[],\"Left\":[{\"id\":\"A\",\"label\":\"A\",\"type\":\"foundation.thermal.thermal\"}],\"Right\":[{\"id\":\"B\",\"label\":\"B\",\"type\":\"foundation.thermal.thermal\"}],\"Top\":[{\"id\":\"Na\",\"label\":\"Na\",\"type\":\"input\"},{\"id\":\"Nb\",\"label\":\"Nb\",\"type\":\"input\"}]}"
  nTraysXnRacks : fl_lib/Physical Signals/Sources/PS Constant  constant=nTrays*nRacks
  one : fl_lib/Physical Signals/Sources/PS Constant  constant=1
  U_gpu : PMIOPort  Side=Left
  U_cpu : PMIOPort  Port=2  Side=Left
  Ha : PMIOPort  Port=3  Side=Left
  P : PMIOPort  Port=4  Side=Right
  T_gpu : PMIOPort  Port=5  Side=Right
  T_cpu : PMIOPort  Port=6  Side=Right
  Hc : PMIOPort  Port=7  Side=Right
  connections:
  Server Tray/LConn1 -- U_gpu/RConn1
  TMamb/LConn1 -- Ha/RConn1
  Server Tray/RConn2 -- T_gpu/RConn1
  TMcdu/RConn1 -- Hc/RConn1
  Server Tray/LConn2 -- U_cpu/RConn1
  Server Tray/RConn3 -- T_cpu/RConn1
  one/RConn1 -- TMcdu/LConn3 -- TMamb/LConn2
  Server Tray/RConn4 -- TMcdu/LConn1
  Server Tray/LConn3 -- TMamb/RConn1
  nTraysXnRacks/RConn1 -- PS Product/LConn1 -- TMcdu/LConn2 -- TMamb/LConn3
  Server Tray/RConn1 -- PS Product/LConn2
  PS Product/RConn1 -- P/RConn1

== system AirCooledDataCenterTemperatureProfile/DataCenter/Air Cooled PDU Assembly 2/Rack Air Cooling ==
  Flowrate vs Eff : fl_lib/Physical Signals/Lookup Tables/PS Lookup Table (1D)  x=flowVec m^3/s  f=fanEffVec  interp_method=simscape.enum.interpolation.linear  extrap_method=simscape.enum.extrapolation.nearest
  Flowrate vs Pressure Drop : fl_lib/Physical Signals/Lookup Tables/PS Lookup Table (1D)  x=flowVec m^3/s  f=prDropVec Pa  interp_method=simscape.enum.interpolation.linear  extrap_method=simscape.enum.extrapolation.nearest
  MaxFlowrate : fl_lib/Physical Signals/Functions/PS Gain  gain=max(flowVec) m^3/s
  PS Divide : fl_lib/Physical Signals/Functions/PS Divide
  PS Product : fl_lib/Physical Signals/Functions/PS Product
  PS Product1 : fl_lib/Physical Signals/Functions/PS Product
  PS Saturation : fl_lib/Physical Signals/Nonlinear Operators/PS Saturation  upper_limit=1  lower_limit=0  ZeroCross=true
  Q : Subsystem
  dT : Subsystem
      settings: PortSchema="{\"entries\":[{\"content\":{\"sides\":[{\"content\":{\"connectorIds\":[\"LConn1\"]},\"type\":\"ConnectorPlacement.EquallySpacedRectSide\",\"uuid\":\"24179a54-9ef9-408d-b9e3-71fcbe48c3e7\"},{\"content\":{\"connectorIds\":[\"RConn1\"],\"side\":\"RIGHT\"},\"type\":\"ConnectorPlacement.EquallySpacedRectSide\",\"uuid\":\"9ef8b705-2d29-4693-9aa8-2fb03fb72ba0\"},{\"content\":{\"side\":\"TOP\"},\"type\":\"ConnectorPlacement.EquallySpacedRectSide\",\"uuid\":\"67fd6558-0b74-41b6-9065-c50d20bb7de5\"},{\"content\":{\"connectorIds\":[\"RConn2\"],\"side\":\"BOTTOM\"},\"type\":\"ConnectorPlacement.EquallySpacedRectSide\",\"uuid\":\"dead0843-c913-4c5f-8840-2a92db603c86\"}]},\"type\":\"ConnectorPlacement.EquallySpacedConnector\",\"uuid\":\"734a32c8-d564-4672-86f6-d3d1b9b4eb6d\"}],\"packageUris\":[\"http://schema.mathworks.com/mf0/Connector/R2020b\"],\"version\":\"1.0\"}"
  m_dot_Cp : Subsystem
      settings: PortSchema="{\"entries\":[{\"content\":{\"sides\":[{\"content\":{},\"type\":\"ConnectorPlacement.EquallySpacedRectSide\",\"uuid\":\"30dae9bf-ed85-460d-bbc0-602f54b59459\"},{\"content\":{\"side\":\"RIGHT\"},\"type\":\"ConnectorPlacement.EquallySpacedRectSide\",\"uuid\":\"05907a20-db7b-437b-af9c-28a9e12dbb0f\"},{\"content\":{\"connectorIds\":[\"LConn1\"],\"side\":\"TOP\"},\"type\":\"ConnectorPlacement.EquallySpacedRectSide\",\"uuid\":\"1394250d-0f3a-4d32-aa79-d5be723ed221\"},{\"content\":{\"connectorIds\":[\"RConn1\"],\"side\":\"BOTTOM\"},\"type\":\"ConnectorPlacement.EquallySpacedRectSide\",\"uuid\":\"8d71629e-6ed3-4a45-8875-f0ad6e4187c2\"}]},\"type\":\"ConnectorPlacement.EquallySpacedConnector\",\"uuid\":\"77e9989b-961e-42ca-a28b-c98959ddb965\"}],\"packageUris\":[\"http://schema.mathworks.com/mf0/Connector/R2020b\"],\"version\":\"1.0\"}"
  numFans : fl_lib/Physical Signals/Sources/PS Constant  constant=nFans
  C : PMIOPort  Side=Left
  S : PMIOPort  Port=2  Side=Left
  H : PMIOPort  Port=3  Side=Right
  P : PMIOPort  Port=4  Side=Right
  connections:
  Flowrate vs Eff/LConn1 -- PS Product/LConn2 -- Flowrate vs Pressure Drop/LConn1 -- MaxFlowrate/RConn1 -- m_dot_Cp/RConn1
  PS Product1/LConn2 -- PS Product/RConn1
  PS Saturation/LConn1 -- S/RConn1
  PS Product1/RConn1 -- PS Divide/LConn1
  PS Divide/LConn2 -- Flowrate vs Eff/RConn1
  PS Divide/RConn1 -- P/RConn1
  PS Saturation/RConn1 -- MaxFlowrate/LConn1
  numFans/RConn1 -- PS Product1/LConn1
  PS Product/LConn1 -- Flowrate vs Pressure Drop/RConn1
  Q/RConn1 -- dT/RConn1 -- H/RConn1
  dT/LConn1 -- C/RConn1
  Q/LConn1 -- dT/RConn2
  m_dot_Cp/LConn1 -- Q/LConn2
